simulink model "counter_verify"  (R2017a)
settings: Solver=FixedStepDiscrete  StartTime=0.0  StopTime=10.0  RelTol=1e-3
libraries: sldvlib x1
settings Model: Creator=rober  LastModifiedBy=rober

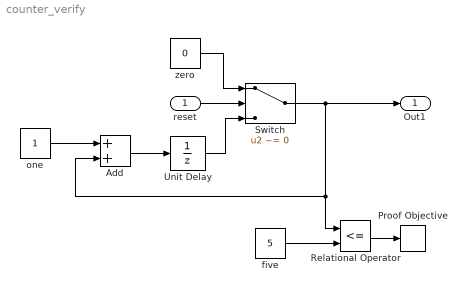
== system counter_verify ==
  reset : Inport  OutDataTypeStr=boolean
  Add : Sum  OutDataTypeStr=uint32
  Proof Objective : sldvlib/Objectives and Constraints/Proof Objective  enabled=on  customAVTBlockType=Proof Objective  intervals=true  dispValues=on  outEnabled=off  enableStopSim=off
      settings: AttributesFormatString=%<intervals>  SourceProductName=Simulink Design Verifier  SourceProductBaseCode=DV
  Relational Operator : RelationalOperator  Operator=<=  OutDataTypeStr=boolean  RndMeth=Simplest
  Switch : Switch  Criteria=u2 ~= 0
  Unit Delay : UnitDelay  SampleTime=-1
  five : Constant  Value=5  OutDataTypeStr=uint32
  one : Constant  OutDataTypeStr=uint32
  zero : Constant  Value=0  OutDataTypeStr=uint32
  Out1 : Outport
  wires:
  Add/1 -> Unit Delay/1
  one/1 -> Add/1
  Switch/1 -> Relational Operator/1, Add/2, Out1/1
  zero/1 -> Switch/1
  Unit Delay/1 -> Switch/3
  reset/1 -> Switch/2
  five/1 -> Relational Operator/2
  Relational Operator/1 -> Proof Objective/1
